simulink model "model"  (R2014a)
settings: Solver=ode45  StartTime=0.0  StopTime=10.0  RelTol=1e-3
undefined symbols (not defined in the file or in its folder): theta1, theta2
settings Model: Creator=mateusz  LastModifiedBy=mateusz

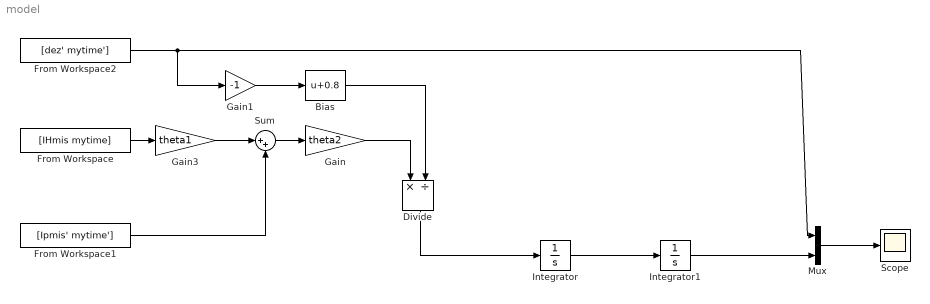
== system model ==
  Bias : Bias  Bias=0.8
  Divide : Product  Inputs=*/
  From Workspace : FromWorkspace  VariableName=[IHmis mytime]  SampleTime=0
  From Workspace1 : FromWorkspace  VariableName=[Ipmis' mytime']  SampleTime=0
  From Workspace2 : FromWorkspace  VariableName=[dez' mytime']  SampleTime=0
  Gain : Gain  Gain=theta2
  Gain1 : Gain  Gain=-1
  Gain3 : Gain  Gain=theta1
  Integrator : Integrator
  Integrator1 : Integrator
  Mux : Mux  Inputs=2
  Scope : Scope
  Sum : Sum  Inputs=|++
  wires:
  Integrator/1 -> Integrator1/1
  Integrator1/1 -> Mux/2
  From Workspace2/1 -> Gain1/1, Mux/1
  Mux/1 -> Scope/1
  From Workspace/1 -> Gain3/1
  From Workspace1/1 -> Sum/2
  Sum/1 -> Gain/1
  Gain3/1 -> Sum/1
  Gain/1 -> Divide/1
  Divide/1 -> Integrator/1
  Gain1/1 -> Bias/1
  Bias/1 -> Divide/2
